simulink model "DCMotor_ver3"  (R2024b)
settings: Solver=VariableStepAuto  StartTime=0.0  StopTime=10.0  RelTol=1e-3
values from neighbouring files (symbols this model uses):
  J = 0.05    [main.m]
  Kii = Kpi/Tii    (= 250)    [main.m]
  Kiw = Kpw/Tiw    (= 10.4166666667)    [main.m]
  kphi = 1.5    [main.m]
  Kpi = Tii/(2*(1/R)*T_p)    (= 2.5)    [main.m]
  Kpw = J/(2*kphi*2*T_p)    (= 0.833333333333)    [main.m]
  L = 0.05    [main.m]
  OM = 50    [main.m]
  R = 5    [main.m]
settings Model: Creator=Student  LastModifiedBy=limok
settings ModelReferenceCC: EnableRefExpFcnMdlSchedulingChecks=on
settings RTWCC: GPUComputeCapability=3.5

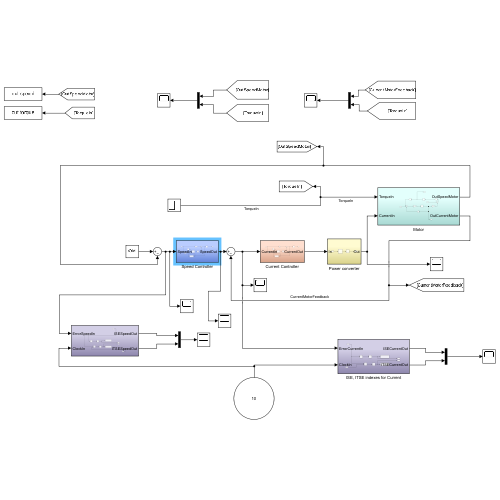
[thumbnail: Simulink's stored preview of the top-level diagram]
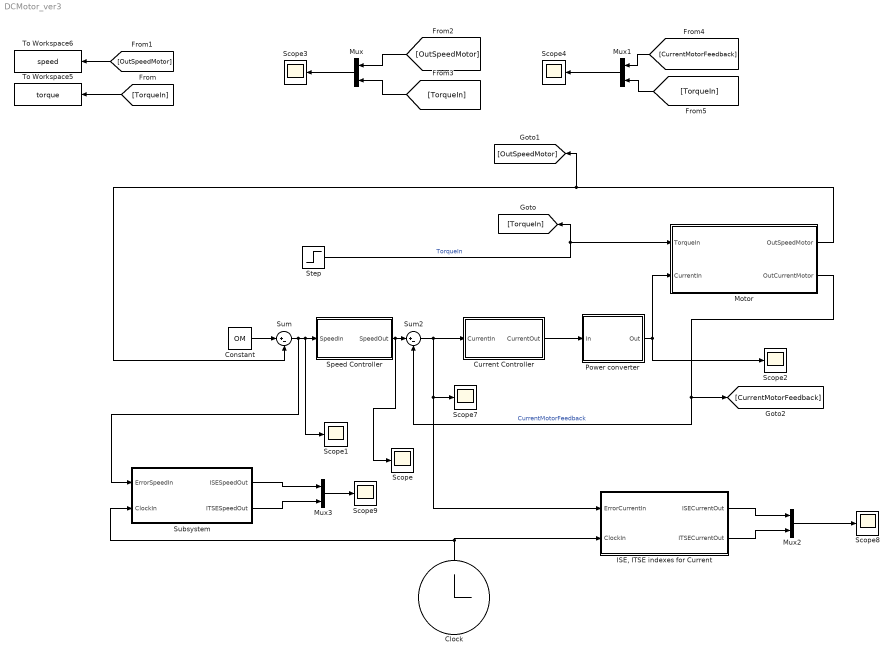
== system DCMotor_ver3 ==
  Clock : Clock
  Constant : Constant  Value=OM
  Current Controller : Subsystem
  "ISE, ITSE indexes for Current" : Subsystem
  Motor : Subsystem
  Mux{,1..3} (4 alike) : Mux  Inputs=2
  Power converter : Subsystem
  Scope{,1..4,7..9} (8 alike) : Scope
  Speed Controller : Subsystem
  Step : Step  SampleTime=0
  Subsystem : Subsystem
  Sum : Sum  Inputs=|+-
  Sum2 : Sum  Inputs=|+-
  To Workspace5 : ToWorkspace  VariableName=torque  SaveFormat=Timeseries  SampleTime=-1
  To Workspace6 : ToWorkspace  VariableName=speed  SaveFormat=Timeseries  SampleTime=-1
  wires:
  Step/1 -> Motor/1(TorqueIn), [TorqueIn]  "TorqueIn"
  Power converter/1(Out) -> Motor/2(CurrentIn), Scope2/1
  Motor/2(OutCurrentMotor) -> Sum2/2, [CurrentMotorFeedback]  "CurrentMotorFeedback"
  Constant/1 -> Sum/1
  Speed Controller/1(SpeedOut) -> Scope/1, Sum2/1
  Sum2/1 -> Current Controller/1(CurrentIn), "ISE, ITSE indexes for Current"/1(ErrorCurrentIn), Scope7/1
  Mux/1 -> Scope3/1
  Mux1/1 -> Scope4/1
  Clock/1 -> "ISE, ITSE indexes for Current"/2(ClockIn), Subsystem/2(ClockIn)
  Mux2/1 -> Scope8/1
  Sum/1 -> Scope1/1, Speed Controller/1(SpeedIn), Subsystem/1(ErrorSpeedIn)
  Mux3/1 -> Scope9/1
  Current Controller/1(CurrentOut) -> Power converter/1(In)
  "ISE, ITSE indexes for Current"/2(ITSECurrentOut) -> Mux2/2
  Subsystem/1(ISESpeedOut) -> Mux3/1
  Subsystem/2(ITSESpeedOut) -> Mux3/2
  "ISE, ITSE indexes for Current"/1(ISECurrentOut) -> Mux2/1
  [OutSpeedMotor] -> To Workspace6/1
  [TorqueIn] -> To Workspace5/1
  [OutSpeedMotor] -> Mux/1
  [TorqueIn] -> Mux/2
  [CurrentMotorFeedback] -> Mux1/1
  [TorqueIn] -> Mux1/2
  Motor/1(OutSpeedMotor) -> Sum/2, [OutSpeedMotor]

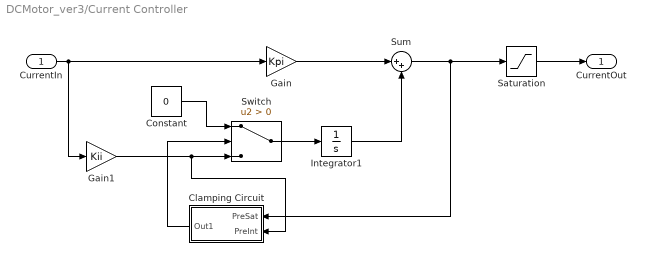
== system DCMotor_ver3/Current Controller ==
  CurrentIn : Inport
  Clamping Circuit : Subsystem
  Constant : Constant  Value=0
  Gain : Gain  Gain=Kpi
  Gain1 : Gain  Gain=Kii
  Integrator1 : Integrator
  Saturation : Saturate  UpperLimit=250  LowerLimit=-250
  Sum : Sum  Inputs=|++
  Switch : Switch  Criteria=u2 > Threshold  SaturateOnIntegerOverflow=off  InputSameDT=off
  CurrentOut : Outport
  wires:
  CurrentIn/1 -> Gain/1, Gain1/1
  Gain/1 -> Sum/1
  Saturation/1 -> CurrentOut/1
  Constant/1 -> Switch/1
  Clamping Circuit/1(Out1) -> Switch/2
  Sum/1 -> Clamping Circuit/1(PreSat), Saturation/1
  Integrator1/1 -> Sum/2
  Gain1/1 -> Clamping Circuit/2(PreInt), Switch/3
  Switch/1 -> Integrator1/1

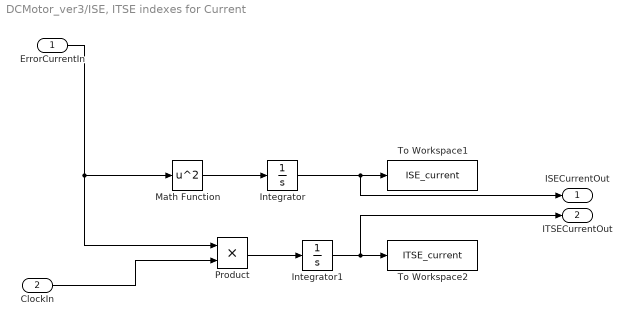
== system DCMotor_ver3/ISE, ITSE indexes for Current ==
  ErrorCurrentIn : Inport
  ClockIn : Inport  Port=2
  Integrator : Integrator
  Integrator1 : Integrator
  Math Function : Math  Operator=square
  Product : Product
  To Workspace1 : ToWorkspace  VariableName=ISE_current  SaveFormat=Timeseries  SampleTime=-1
  To Workspace2 : ToWorkspace  VariableName=ITSE_current  SaveFormat=Timeseries  SampleTime=-1
  ISECurrentOut : Outport
  ITSECurrentOut : Outport  Port=2
  wires:
  Integrator/1 -> ISECurrentOut/1, To Workspace1/1
  Integrator1/1 -> ITSECurrentOut/1, To Workspace2/1
  ErrorCurrentIn/1 -> Math Function/1, Product/1
  ClockIn/1 -> Product/2
  Product/1 -> Integrator1/1
  Math Function/1 -> Integrator/1

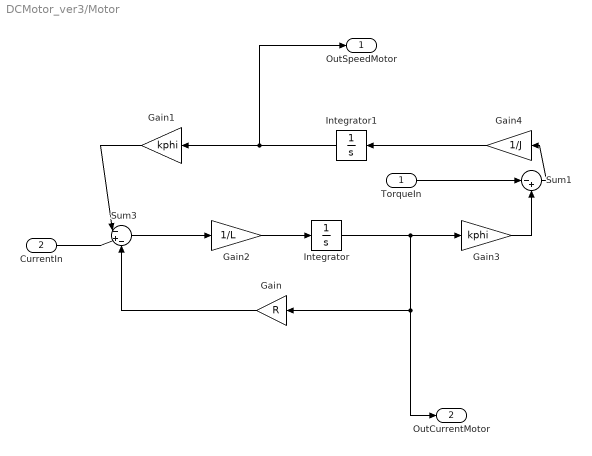
== system DCMotor_ver3/Motor ==
  TorqueIn : Inport
  CurrentIn : Inport  Port=2
  Gain : Gain  Gain=R
  Gain1 : Gain  Gain=kphi
  Gain2 : Gain  Gain=1/L
  Gain3 : Gain  Gain=kphi
  Gain4 : Gain  Gain=1/J
  Integrator : Integrator
  Integrator1 : Integrator
  Sum1 : Sum  Inputs=|-+
  Sum3 : Sum  Inputs=|-+-
  OutSpeedMotor : Outport
  OutCurrentMotor : Outport  Port=2
  wires:
  Integrator1/1 -> OutSpeedMotor/1, Gain1/1
  Gain2/1 -> Integrator/1
  Gain1/1 -> Sum3/1
  Gain/1 -> Sum3/3
  Gain3/1 -> Sum1/2
  Integrator/1 -> Gain3/1, OutCurrentMotor/1, Gain/1
  Sum1/1 -> Gain4/1
  Sum3/1 -> Gain2/1
  CurrentIn/1 -> Sum3/2
  TorqueIn/1 -> Sum1/1
  Gain4/1 -> Integrator1/1

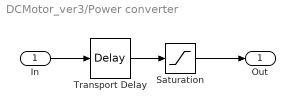
== system DCMotor_ver3/Power converter ==
  In : Inport
  Saturation : Saturate  UpperLimit=250  LowerLimit=-250
  Transport Delay : TransportDelay  DelayTime=0.01
  Out : Outport
  wires:
  Transport Delay/1 -> Saturation/1
  In/1 -> Transport Delay/1
  Saturation/1 -> Out/1

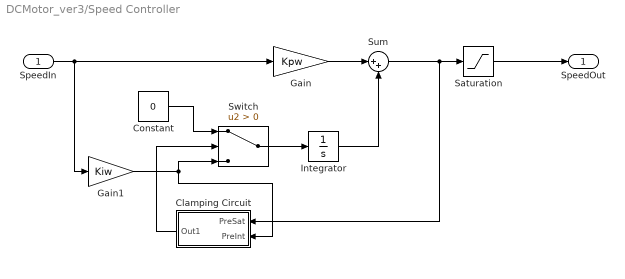
== system DCMotor_ver3/Speed Controller ==
  SpeedIn : Inport
  Clamping Circuit : Subsystem
  Constant : Constant  Value=0
  Gain : Gain  Gain=Kpw
  Gain1 : Gain  Gain=Kiw
  Integrator : Integrator
  Saturation : Saturate  UpperLimit=7  LowerLimit=-7
  Sum : Sum  Inputs=|++
  Switch : Switch  Criteria=u2 > Threshold  SaturateOnIntegerOverflow=off  InputSameDT=off
  SpeedOut : Outport
  wires:
  SpeedIn/1 -> Gain1/1, Gain/1
  Gain/1 -> Sum/1
  Sum/1 -> Clamping Circuit/1(PreSat), Saturation/1
  Integrator/1 -> Sum/2
  Constant/1 -> Switch/1
  Gain1/1 -> Switch/3, Clamping Circuit/2(PreInt)
  Switch/1 -> Integrator/1
  Clamping Circuit/1(Out1) -> Switch/2
  Saturation/1 -> SpeedOut/1

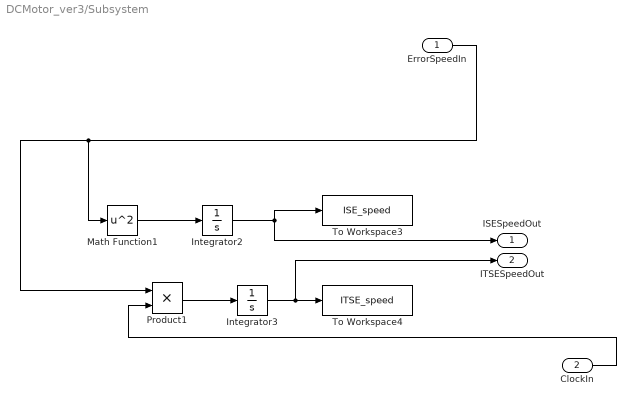
== system DCMotor_ver3/Subsystem ==
  ErrorSpeedIn : Inport
  ClockIn : Inport  Port=2
  Integrator2 : Integrator
  Integrator3 : Integrator
  Math Function1 : Math  Operator=square
  Product1 : Product
  To Workspace3 : ToWorkspace  VariableName=ISE_speed  SaveFormat=Timeseries  SampleTime=-1
  To Workspace4 : ToWorkspace  VariableName=ITSE_speed  SaveFormat=Timeseries  SampleTime=-1
  ISESpeedOut : Outport
  ITSESpeedOut : Outport  Port=2
  wires:
  Integrator3/1 -> ITSESpeedOut/1, To Workspace4/1
  ClockIn/1 -> Product1/2
  Math Function1/1 -> Integrator2/1
  Integrator2/1 -> ISESpeedOut/1, To Workspace3/1
  ErrorSpeedIn/1 -> Math Function1/1, Product1/1
  Product1/1 -> Integrator3/1

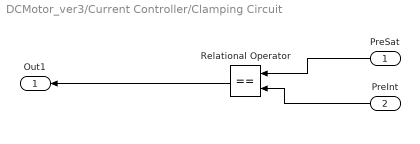
== system DCMotor_ver3/Current Controller/Clamping Circuit ==
  PreSat : Inport
  PreInt : Inport  Port=2
  Relational Operator : RelationalOperator  Operator===  OutDataTypeStr=boolean  RndMeth=Simplest  InputSameDT=off
  Out1 : Outport
  wires:
  PreSat/1 -> Relational Operator/1
  PreInt/1 -> Relational Operator/2
  Relational Operator/1 -> Out1/1

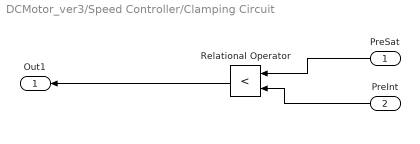
== system DCMotor_ver3/Speed Controller/Clamping Circuit ==
  PreSat : Inport
  PreInt : Inport  Port=2
  Relational Operator : RelationalOperator  Operator=<  OutDataTypeStr=boolean  RndMeth=Simplest  InputSameDT=off
  Out1 : Outport
  wires:
  PreSat/1 -> Relational Operator/1
  PreInt/1 -> Relational Operator/2
  Relational Operator/1 -> Out1/1
